simulink model "celsiusConverter_StevenJohnson"  (R2025b)
settings: Solver=VariableStepAuto  StartTime=0.0  StopTime=10.0  RelTol=1e-3
libraries: aerolibconvert2 x3

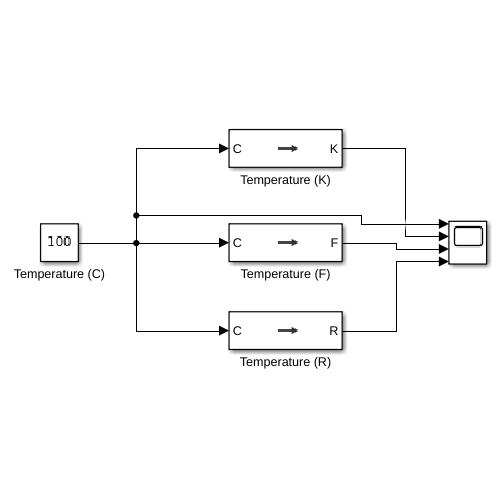
[thumbnail: Simulink's stored preview of the top-level diagram]
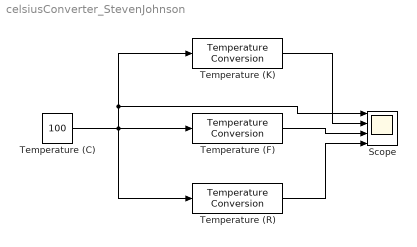
== system celsiusConverter_StevenJohnson ==
  Scope : Scope  NumInputPorts=4
      settings: ActiveDisplayYMinimum=-73.418736505046809  ActiveDisplayYMaximum=681.77561818245408  YLabel=Temperature (R,F,K,C)
  Temperature (C) : Constant  Value=100  SampleTime=0
  Temperature (F) : aerolibconvert2/Temperature Conversion  IU=C  OU=F
  Temperature (K) : aerolibconvert2/Temperature Conversion  IU=C  OU=K
  Temperature (R) : aerolibconvert2/Temperature Conversion  IU=C  OU=R
  wires:
  Temperature (C)/1 -> Temperature (R)/1, Temperature (F)/1, Temperature (K)/1, Scope/1
  Temperature (F)/1 -> Scope/3
  Temperature (R)/1 -> Scope/4
  Temperature (K)/1 -> Scope/2
